simulink model "EPS_newest_not_easy"  (R2022b)
settings: Solver=VariableStepAuto  StartTime=0.0  StopTime=10.0  RelTol=1e-3  AbsTol=1e-3  EnableMultiTasking=on
undefined symbols (not defined in the file): B1, Br, Bsw, CFr, Ef, Jeq, Jsw, Ksc, Ktr, Mr, Rp
settings Model: Creator=ASUS  LastModifiedBy=ASUS
settings SolverCC: AutoScaleAbsTol=off  AlgebraicLoopSolver=TrustRegion  MaxZcPerStep=1
settings DataIOCC: LimitDataPoints=on  MaxDataPoints=10000
settings OptimizationCC: LifeSpan=inf
settings DebuggingCC: UnconnectedInputMsg=warning  UnconnectedOutputMsg=warning  UnconnectedLineMsg=warning  AllowSymbolicDim=off  SFUnexpectedBacktrackingDiag=warning  SFNoUnconditionalDefaultTransitionDiag=warning  SFExecutionAtInitializationDiag=none  SFMachineParentedDataDiag=warning  ArithmeticOperatorsInVariantConditions=warning
settings ModelReferenceCC: EnableRefExpFcnMdlSchedulingChecks=on
settings SFSimCC: SimUseLocalCustomCode=off  CustomCodeUndefinedFunction=UseInterfaceOnly
settings RTWCC: RTWUseLocalCustomCode=off  DLArmComputeVersion=19.05
settings CodeAppCC: StateflowObjectComments=on
settings GRTTargetCC: TargetLangStandard=C89/C90 (ANSI)
settings ConfigComp: CovMetricSettings=dw  CovSaveCumulativeToWorkspaceVar=on  CovSaveSingleToWorkspaceVar=on  CovExternalEMLEnable=off  CovSFcnEnable=off
settings SimscapeCC: SimscapeLogType=all  SimscapeLogSimulationStatistics=on  SimscapeLogDataHistory=10000

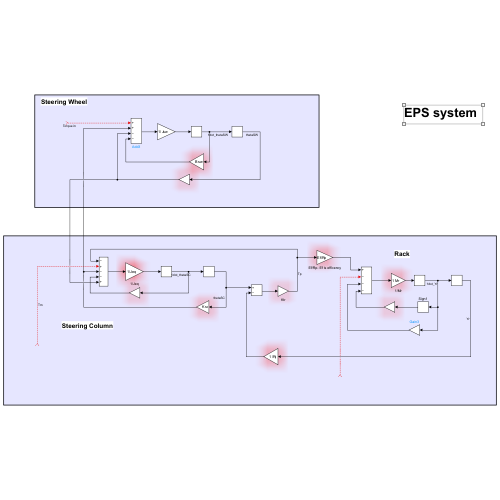
[thumbnail: Simulink's stored preview of the top-level diagram]
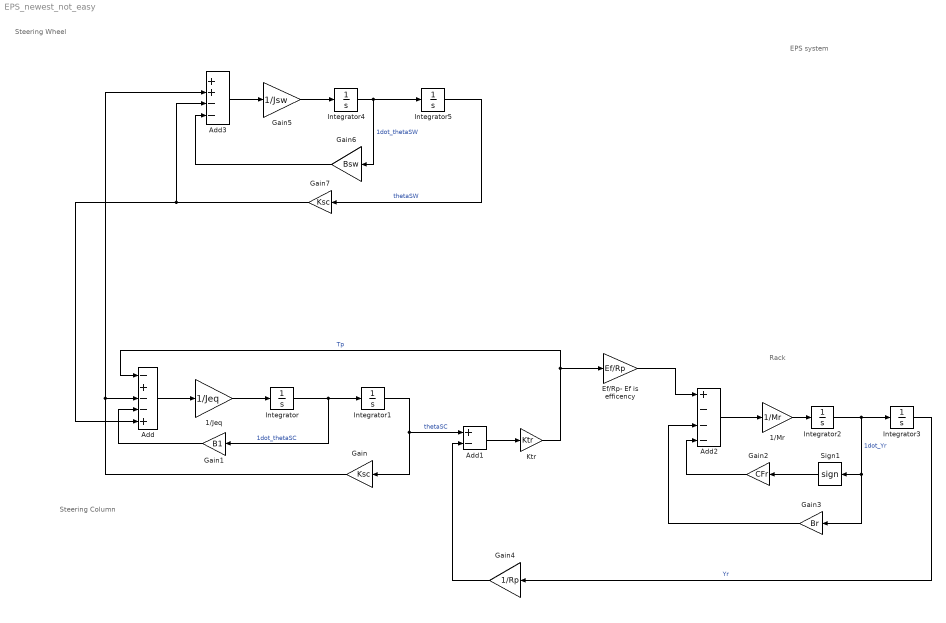
== system EPS_newest_not_easy ==
  note: EPS system
  note: Rack
  note: Steering Column
  note: Steering Wheel
  1/Jeq : Gain  Gain=1/Jeq
  1/Mr : Gain  Gain=1/Mr
  Add : Sum  Inputs=-+--+
  Add1 : Sum  Inputs=+-
  Add2 : Sum  Inputs=+---
  Add3 : Sum  Inputs=++--
  Ef/Rp- Ef is efficency : Gain  Gain=Ef/Rp
  Gain : Gain  Gain=Ksc
  Gain1 : Gain  Gain=B1
  Gain2 : Gain  Gain=CFr
  Gain3 : Gain  Gain=Br
  Gain4 : Gain  Gain=1/Rp
  Gain5 : Gain  Gain=1/Jsw
  Gain6 : Gain  Gain=Bsw
  Gain7 : Gain  Gain=Ksc
  Integrator{,1..5} (6 alike) : Integrator
  Ktr : Gain  Gain=Ktr
  Sign1 : Signum
  wires:
  Add/1 -> 1/Jeq/1
  1/Jeq/1 -> Integrator/1
  Integrator/1 -> Gain1/1, Integrator1/1  "1dot_thetaSC"
  Integrator1/1 -> Add1/1, Gain/1  "thetaSC"
  Gain/1 -> Add3/2, Add/3
  Gain1/1 -> Add/4
  ? -> Add/2  "Tm"
  Add1/1 -> Ktr/1
  Ktr/1 -> Ef/Rp- Ef is efficency/1, Add/1  "Tp"
  Ef/Rp- Ef is efficency/1 -> Add2/1
  Add2/1 -> 1/Mr/1
  1/Mr/1 -> Integrator2/1
  Integrator2/1 -> Gain3/1, Sign1/1, Integrator3/1  "1dot_Yr"
  Integrator3/1 -> Gain4/1  "Yr"
  Sign1/1 -> Gain2/1
  Gain2/1 -> Add2/4
  Gain3/1 -> Add2/3
  ? -> Add2/2
  Gain4/1 -> Add1/2
  ? -> Add3/1  "Torque in"
  Add3/1 -> Gain5/1
  Gain5/1 -> Integrator4/1
  Integrator4/1 -> Gain6/1, Integrator5/1  "1dot_thetaSW"
  Integrator5/1 -> Gain7/1  "thetaSW"
  Gain6/1 -> Add3/4
  Gain7/1 -> Add/5, Add3/3
